simulink model "serialCommTest"  (R2020a)
settings: Solver=FixedStepAuto  StartTime=0.0  StopTime=10.0  FixedStep=1e-3  RelTol=1e-3  EnableMultiTasking=on
libraries: frdmk64flib x5, etargetslib x2
settings Model: ExtModeTrigDuration=5  Creator=emily  LastModifiedBy=emily
settings OptimizationCC: EnhancedBackFolding=on  PassReuseOutputArgsAs=Individual arguments  ZeroExternalMemoryAtStartup=off  ZeroInternalMemoryAtStartup=off  MaxStackSize=64  OptimizeBlockOrder=speed  DifferentSizesBufferReuse=on  OptimizationCustomize=off  EfficientTunableParamExpr=on
settings DebuggingCC: ParameterTunabilityLossMsg=error
settings HardwareCC: ProdBitPerPointer=32  ProdBitPerSizeT=32  ProdBitPerPtrDiffT=32  ProdLargestAtomicInteger=Long  ProdLargestAtomicFloat=Double  ProdWordSize=32  ProdHWDeviceType=ARM Compatible->ARM Cortex
settings SFSimCC: MATLABDynamicMemAlloc=off
settings RTWCC: SystemTargetFile=ert.tlc  HardwareBoard=NXP FRDM-K64F  TemplateMakefile=ert_default_tmf  Toolchain=GNU Tools for ARM Embedded Processors
settings CodeAppCC: ForceParamTrailComments=on  IgnoreCustomStorageClasses=off  OperatorAnnotations=on  SimulinkDataObjDesc=on  SFDataObjDesc=on  InsertBlockDesc=on

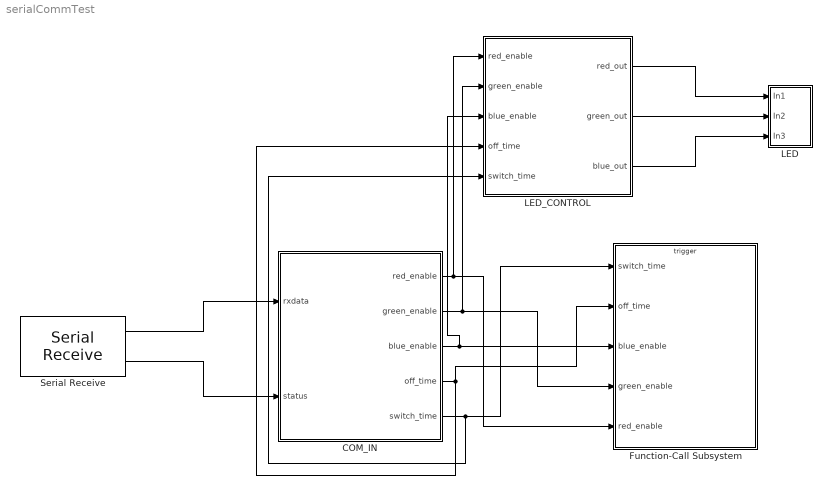
== system serialCommTest ==
  COM_IN : Stateflow chart  TreatAsAtomicUnit=on
  Function-Call Subsystem : Subsystem  TreatAsAtomicUnit=on
  LED : Subsystem
  LED_CONTROL : Stateflow chart  TreatAsAtomicUnit=on
  Serial Receive : frdmk64flib/Serial Receive  SCIModule=0  Baudrate=uint32(9600)  Parity=None  StopBits=1  HardwareFlowControl=None  ByteOrder=LittleEndian  DataType=uint8  DataLength=11  BlockingMode=off  OutputStatus=on  SampleTime=-1
  wires:
  COM_IN/1(red_enable) -> LED_CONTROL/1(red_enable), Function-Call Subsystem/5(red_enable)
  COM_IN/2(green_enable) -> LED_CONTROL/2(green_enable), Function-Call Subsystem/4(green_enable)
  COM_IN/3(blue_enable) -> LED_CONTROL/3(blue_enable), Function-Call Subsystem/3(blue_enable)
  COM_IN/4(off_time) -> LED_CONTROL/4(off_time), Function-Call Subsystem/2(off_time)
  COM_IN/5(switch_time) -> LED_CONTROL/5(switch_time), Function-Call Subsystem/1(switch_time)
  LED_CONTROL/1(red_out) -> LED/1(In1)
  LED_CONTROL/2(green_out) -> LED/2(In2)
  LED_CONTROL/3(blue_out) -> LED/3(In3)
  Serial Receive/1 -> COM_IN/1(rxdata)
  Serial Receive/2 -> COM_IN/2(status)

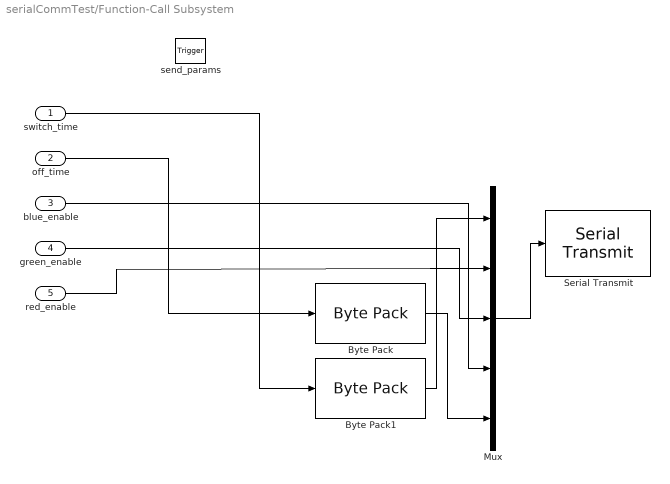
== system serialCommTest/Function-Call Subsystem ==
  switch_time : Inport
  off_time : Inport  Port=2
  blue_enable : Inport  Port=3
  green_enable : Inport  Port=4
  red_enable : Inport  Port=5
  send_params : TriggerPort  TriggerType=function-call  IsSimulinkFunction=on  FunctionName=send_params  VariantControl=Variant
  Byte Pack : etargetslib/Byte Pack  datatypes={'single'}  byteAlign=1
  Byte Pack1 : etargetslib/Byte Pack  datatypes={'uint16'}  byteAlign=1
  Mux : Mux  Inputs=5
  Serial Transmit : frdmk64flib/Serial Transmit  SCIModule=0  Baudrate=uint32(9600)  Parity=None  StopBits=1  HardwareFlowControl=None  ByteOrder=LittleEndian  BlockingMode=on  OutputStatus=off
  wires:
  Mux/1 -> Serial Transmit/1
  Byte Pack/1 -> Mux/5
  switch_time/1 -> Byte Pack1/1
  off_time/1 -> Byte Pack/1
  blue_enable/1 -> Mux/4
  green_enable/1 -> Mux/3
  red_enable/1 -> Mux/2
  Byte Pack1/1 -> Mux/1

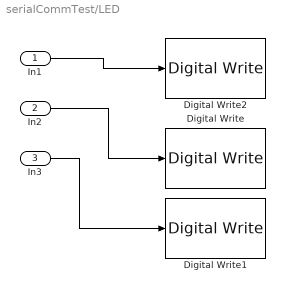
== system serialCommTest/LED ==
  In1 : Inport
  In2 : Inport  Port=2
  In3 : Inport  Port=3
  Digital Write : frdmk64flib/Digital Write  Whichpin=GREEN_LED
  Digital Write1 : frdmk64flib/Digital Write  Whichpin=BLUE_LED
  Digital Write2 : frdmk64flib/Digital Write  Whichpin=RED_LED
  wires:
  In1/1 -> Digital Write2/1
  In2/1 -> Digital Write/1
  In3/1 -> Digital Write1/1

== stateflow chart serialCommTest/LED_CONTROL ==
  state OFF
    entry:
    red_out = false;
    green_out = false;
    blue_out = false;
  state RED_ON
    entry:
    red_out = true;
    green_out = false;
    blue_out = false;
  state BLUE_ON
    entry:
    red_out =false;
    green_out = false;
    blue_out = true;
  state GREEN_ON
    entry:
    red_out = false;
    green_out = true;
    blue_out = false;
  (default) -> OFF
  OFF -> (junction 6) : after(off_time, sec)
  (junction 6) -> RED_ON [order 1] : [red_enable == 1]
  (junction 6) -> (junction 7) [order 2]
  RED_ON -> (junction 7) : after(switch_time,msec)
  (junction 9) -> OFF
  (junction 7) -> (junction 8) [order 2]
  (junction 8) -> (junction 9) [order 2]
  BLUE_ON -> (junction 9) : after(switch_time,msec)
  (junction 7) -> GREEN_ON [order 1] : [green_enable == 1]
  (junction 8) -> BLUE_ON [order 1] : [blue_enable == 1]
  GREEN_ON -> (junction 8) : after(switch_time,msec)
  data: red_enable input uint8; green_enable input uint8; blue_enable input uint8; off_time input single; switch_time input uint16; red_out output boolean; green_out output boolean; blue_out output boolean

== stateflow chart serialCommTest/COM_IN ==
  settings: executeAtInitialization=1
  state SET_PARAM
    entry:
    red_enable = rxdata(3)
    green_enable = rxdata(4);
    blue_enable = rxdata(5);
    off_time = typecast(rxdata(6:9), 'single');
    switch_time = typecast(rxdata(10:11), 'uint16');
  state INITIAL
    entry:
    red_enable = 1;
    green_enable = 1;
    blue_enable = 1;
    off_time = 0.5;
    switch_time = 200;
  state STANDBY
  state ECHO_PARAM
    entry:
    send_params();
  SET_PARAM -> STANDBY
  (junction 9) -> SET_PARAM [order 2] : [rxdata(2) == hex2dec('55')]
  (default) -> INITIAL
  (junction 8) -> STANDBY [order 2]
  INITIAL -> STANDBY
  STANDBY -> (junction 8) : [status == 0]
  (junction 8) -> (junction 9) [order 1] : [rxdata(1) == hex2dec('16')]
  (junction 9) -> ECHO_PARAM [order 1] : [rxdata(2) == hex2dec('22')]
  ECHO_PARAM -> STANDBY
  data: rxdata input uint8; status input uint8; red_enable output uint8; green_enable output uint8; blue_enable output uint8; off_time output single; switch_time output uint16
